simulink model "VDB_ClosedLoop"  (R2026b)
settings: Solver=ode4  StopTime=35  FixedStep=0.02
undefined symbols (not defined in the file or in its folder): sih
libraries: autolibshared x1
settings Model: Creator=Hp  LastModifiedBy=Hp

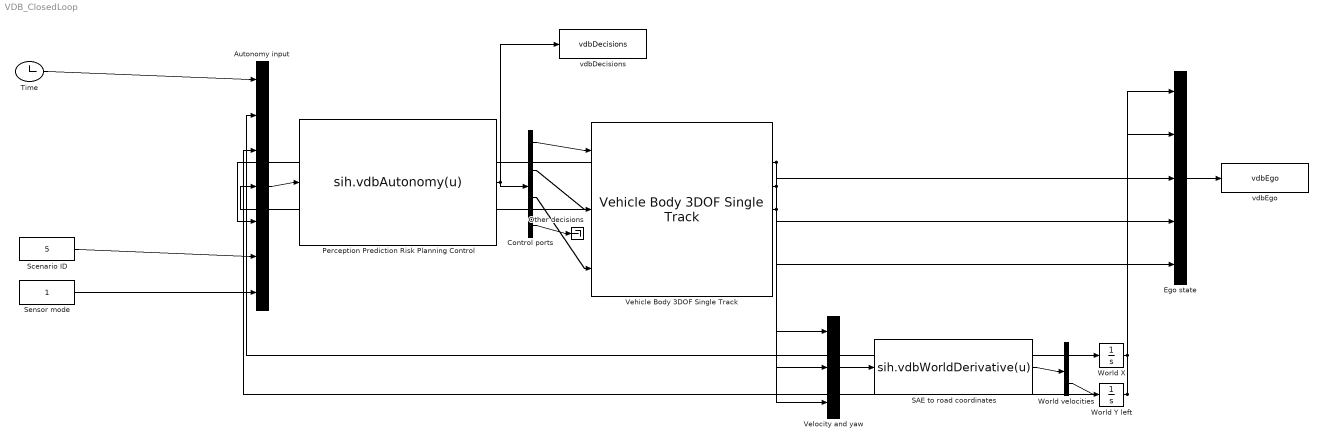
== system VDB_ClosedLoop ==
  Autonomy input : Mux  Inputs=7
  Control ports : Demux  Outputs=[1 1 1 27]
  Ego state : Mux  Inputs=5
  Other decisions : Terminator
  Perception Prediction Risk Planning Control : MATLABFcn  MATLABFcn=sih.vdbAutonomy(u)  OutputDimensions=30  SampleTime=0.1
  SAE to road coordinates : MATLABFcn  MATLABFcn=sih.vdbWorldDerivative(u)  OutputDimensions=2  SampleTime=0.02
  Scenario ID : Constant  Value=5
  Sensor mode : Constant
  Time : Clock
  Vehicle Body 3DOF Single Track : autolibshared/Vehicle Body 3DOF Single Track  trackMode=Single (bicycle)  inputMode=External longitudinal forces  frontSteerMode=on  rearSteerMode=off  extFMode=off  htchFMode=off  extMMode=off  htchMMode=off  windMode=off  extTamb=off  muMode=off  extGndPlnElev=off  extGndPlnRoll=off  extGndPlnPitch=off  extGndPlnDCM=off  extXo=off  extxdoto=off  extYo=off  extydoto=off  extpsio=off  extro=off  aMode=2  NF=2  NR=2  m=2000  a=1.35  b=1.35  h=0.35  dh=1  hh=0.2  X_o=0  xdot_o=0  d=0  hl=0  w=[1.4,1.4]  CalphaMode=Constant  sigmaMode=on  sigma_f=.1  sigma_r=.1  Cy_f=12e3  Cy_r=11e3  Cy_f_data="[1.396121365092108e+04\t4.232462640127975e+04\t6.754894575573687e+04\t8.835784428391886e+04\t1.043551700699839e+05\t1.158335754468729e+05\t1.234691551560788e+05\t1.280575366661118e+05\t1.298126639907242e+05\t1.298126639907242e+05]"  alpha_f_brk=[-0.785, -0.628, -0.471, -0.314, -0.157, 0.000, 0.157, 0.314, 0.471, 0.628, 0.785]  Fz_f_brk="[500\t1.555555555555556e+03\t2.611111111111111e+03\t3.666666666666667e+03\t4.722222222222223e+03\t5.777777777777777e+03\t6.833333333333333e+03\t7.888888888888889e+03\t8.944444444444445e+03\t10000]"  Cy_r_data="[1.396121365092108e+04\t4.232462640127975e+04\t6.754894575573687e+04\t8.835784428391886e+04\t1.043551700699839e+05\t1.158335754468729e+05\t1.234691551560788e+05\t1.280575366661118e+05\t1.298126639907242e+05\t1.298126639907242e+05]"  alpha_r_brk=[-0.785, -0.628, -0.471, -0.314, -0.157, 0.000, 0.157, 0.314, 0.471, 0.628, 0.785]  Fz_r_brk="[500\t1.555555555555556e+03\t2.611111111111111e+03\t3.666666666666667e+03\t4.722222222222223e+03\t5.777777777777777e+03\t6.833333333333333e+03\t7.888888888888889e+03\t8.944444444444445e+03\t10000]"  Fznom=5000  Y_o=0  ydot_o=0  Izz=4000  psi_o=0  r_o=0  Af=2  Cd=.3  Cl=.1  Cpm=.1  beta_w=[0,0.1745,0.3491,0.5236,0.6981,0.8727,1.0472,1.2217,1.3963,1.5708]  Cs=[0.1000,0.1000,0.1000,0.1000,0.1000,0.1000,0.1000,0.1000,0.1000,0.1000]  Cym=[0,0,0.0667,0.1000,0.1333,0.1667,0.2000,0.2333,0.2667,0.3000]  Pabs=101325  Tair=273  g=9.81  mu=1  GndPlnRoll=0  GndPlnPitch=0  GndPlnElev=0  xdot_tol=0.1  Fxtire_sat=7e4  Fytire_sat=7e4  longOff=0  latOff=0  vertOff=0.35  wrapAng=off
  Velocity and yaw : Mux  Inputs=3
  World X : Integrator
  World Y left : Integrator
  World velocities : Demux  Outputs=2
  vdbDecisions : ToWorkspace  VariableName=vdbDecisions  SaveFormat=Timeseries  SampleTime=-1
  vdbEgo : ToWorkspace  VariableName=vdbEgo  SaveFormat=Timeseries  SampleTime=-1
  wires:
  Time/1 -> Autonomy input/1
  World X/1 -> Autonomy input/2, Ego state/1
  World Y left/1 -> Autonomy input/3, Ego state/2
  Vehicle Body 3DOF Single Track/4 -> Autonomy input/4, Velocity and yaw/3, Ego state/3
  Vehicle Body 3DOF Single Track/2 -> Autonomy input/5, Velocity and yaw/1, Ego state/4
  Scenario ID/1 -> Autonomy input/6
  Sensor mode/1 -> Autonomy input/7
  Autonomy input/1 -> Perception Prediction Risk Planning Control/1
  Perception Prediction Risk Planning Control/1 -> Control ports/1, vdbDecisions/1
  Control ports/1 -> Vehicle Body 3DOF Single Track/1
  Control ports/2 -> Vehicle Body 3DOF Single Track/2
  Control ports/3 -> Vehicle Body 3DOF Single Track/3
  Control ports/4 -> Other decisions/1
  Vehicle Body 3DOF Single Track/3 -> Velocity and yaw/2, Ego state/5
  Velocity and yaw/1 -> SAE to road coordinates/1
  SAE to road coordinates/1 -> World velocities/1
  World velocities/1 -> World X/1
  World velocities/2 -> World Y left/1
  Ego state/1 -> vdbEgo/1
